simulink model "Book4131"  (R2019b)
settings: Solver=ode4  StartTime=0  StopTime=10.0  FixedStep=0.001  RelTol=1e-3
settings Model: Creator=xyh  LastModifiedBy=xyh

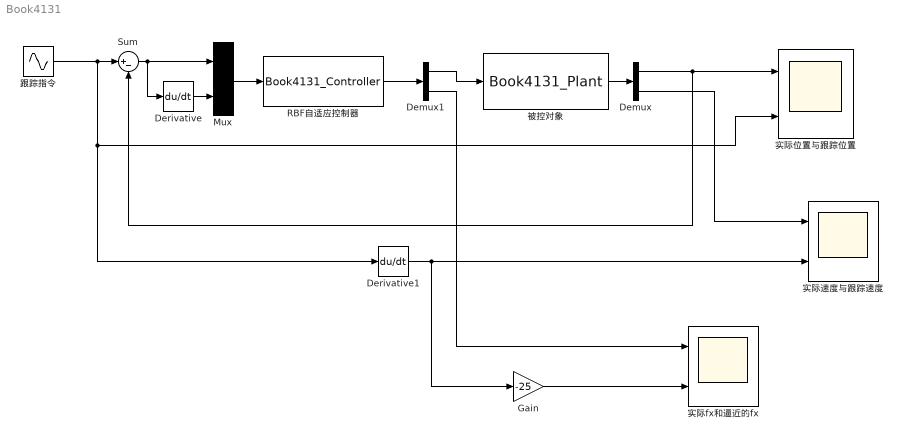
== system Book4131 ==
  Demux : Demux  Outputs=2
  Demux1 : Demux  Outputs=2
  Derivative : Derivative
  Derivative1 : Derivative
  Gain : Gain  Gain=-25
  Mux : Mux  Inputs=2
  RBF自适应控制器 : S-Function  FunctionName=Book4131_Controller  SFunctionDeploymentMode=off  EnableBusSupport=off
  Sum : Sum  Inputs=|+-
  实际fx和逼近的fx : Scope  NumInputPorts=2
  实际位置与跟踪位置 : Scope  NumInputPorts=2
  实际速度与跟踪速度 : Scope  NumInputPorts=2
  被控对象 : S-Function  FunctionName=Book4131_Plant  SFunctionDeploymentMode=off  EnableBusSupport=off
  跟踪指令 : Sin  Amplitude=0.1  SampleTime=0
  wires:
  Demux/1 -> Sum/2, 实际位置与跟踪位置/1
  跟踪指令/1 -> 实际位置与跟踪位置/2, Derivative1/1, Sum/1
  Mux/1 -> RBF自适应控制器/1
  Sum/1 -> Derivative/1, Mux/1
  Derivative/1 -> Mux/2
  被控对象/1 -> Demux/1
  Demux/2 -> 实际速度与跟踪速度/1
  Derivative1/1 -> Gain/1, 实际速度与跟踪速度/2
  RBF自适应控制器/1 -> Demux1/1
  Demux1/1 -> 被控对象/1
  Demux1/2 -> 实际fx和逼近的fx/1
  Gain/1 -> 实际fx和逼近的fx/2
